simulink model "DC_Motor"  (R2017a)
settings: Solver=VariableStepAuto  StartTime=0.0  StopTime=10.0  RelTol=1e-3
settings Model: Creator=uidn7735  LastModifiedBy=uidn7735

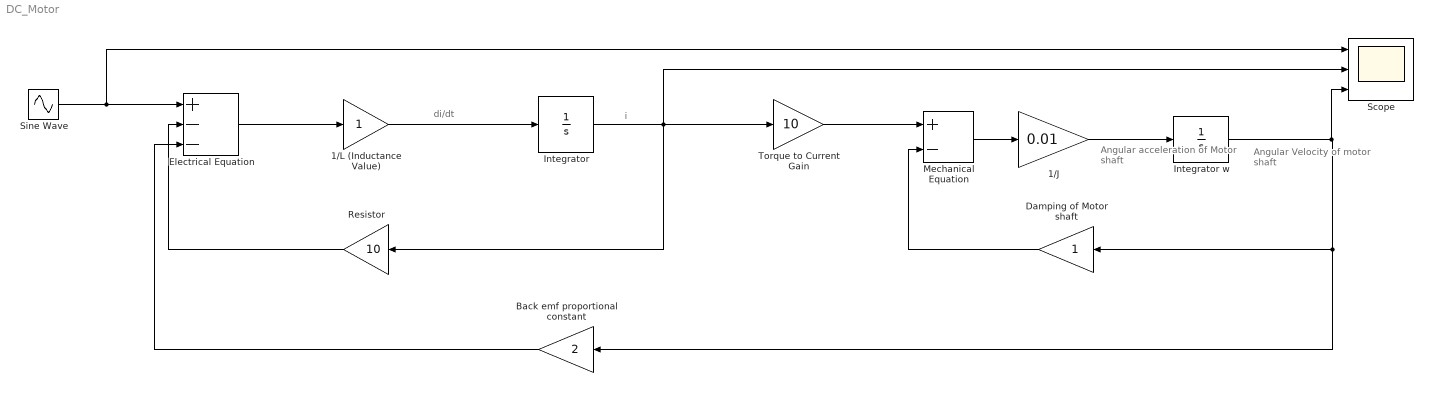
== system DC_Motor ==
  note: Angular Velocity
      | of motor shaft
  note: Angular
      | acceleration
      | of Motor shaft
  note: i
  note: di/dt
  1/J : Gain  Gain=0.01
  1/L (Inductance Value) : Gain
  "Back emf proportional constant " : Gain  Gain=2
  Damping of Motor shaft : Gain
  "Electrical Equation " : Sum  Inputs=+--
  Integrator : Integrator
  Integrator w : Integrator
  "Mechanical Equation " : Sum  Inputs=+-
  Resistor : Gain  Gain=10
  Scope : Scope  NumInputPorts=3
  Sine Wave : Sin  Amplitude=12  SampleTime=0
  Torque to Current Gain : Gain  Gain=10
  wires:
  "Electrical Equation "/1 -> 1/L (Inductance Value)/1
  1/L (Inductance Value)/1 -> Integrator/1
  Integrator/1 -> Scope/2, Resistor/1, Torque to Current Gain/1
  Resistor/1 -> "Electrical Equation "/2
  Torque to Current Gain/1 -> "Mechanical Equation "/1
  "Mechanical Equation "/1 -> 1/J/1
  1/J/1 -> Integrator w/1
  Integrator w/1 -> Scope/3, "Back emf proportional constant "/1, Damping of Motor shaft/1
  Damping of Motor shaft/1 -> "Mechanical Equation "/2
  "Back emf proportional constant "/1 -> "Electrical Equation "/3
  Sine Wave/1 -> Scope/1, "Electrical Equation "/1
